simulink model "IOT_IOT"  (R2024b)
settings: Solver=VariableStepAuto  StartTime=0.0  StopTime=1  RelTol=1e-3
undefined symbols (not defined in the file): Acid, Lead, sigbuilder_block
libraries: spsBatteryLib x81, spsVoltageMeasurementLib x24, spsSeriesRLCBranchLib x23, spsIdealSwitchLib x11, slpidlib x9, spsMosfetLib x9, spsPWMGeneratorDCDCLib x7, spsPWMGenerator2LevelLib x5, spsDiodeLib x4, spsPowerLib x3, spsThreePhaseSeriesRLCLoadLib x2, spsThreePhaseVIMeasurementLib x2
(part 1 of 4)
settings Model: SimulationMode=accelerator  Creator=Jatay  LastModifiedBy=Jatay

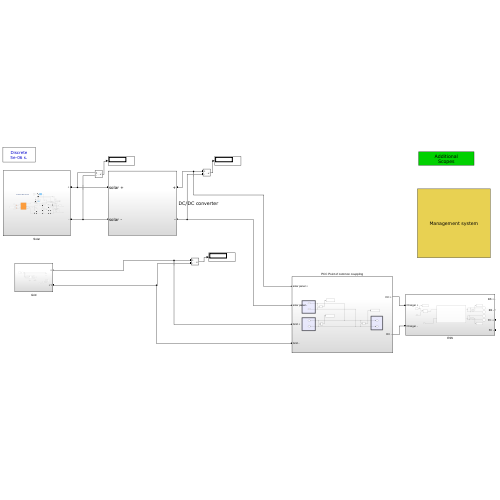
[thumbnail: Simulink's stored preview of the top-level diagram]
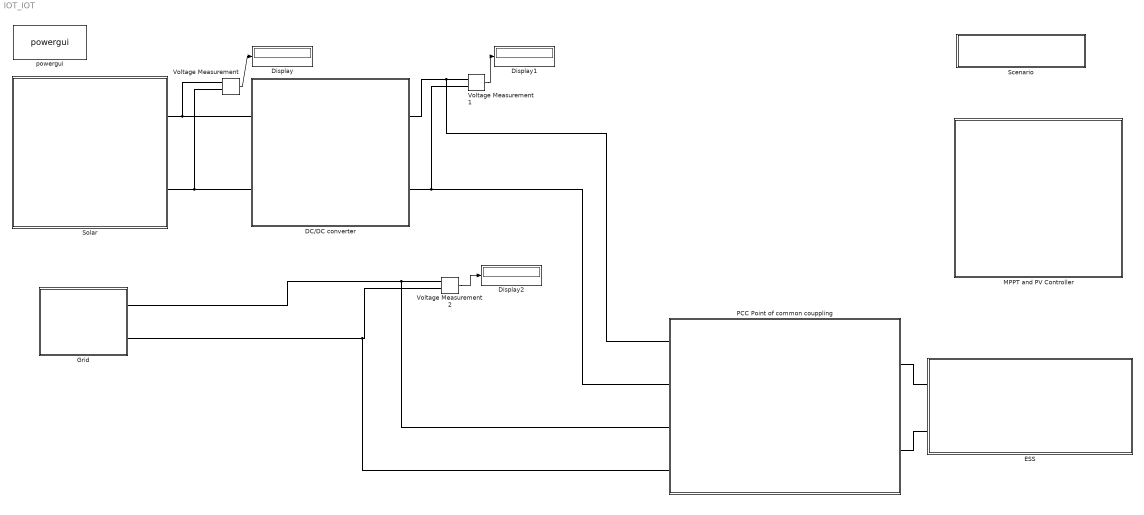
== system IOT_IOT ==
  DC/DC converter : Subsystem
  Display : Display
  Display1 : Display
  Display2 : Display
  ESS : Subsystem
  Grid : Subsystem
  MPPT and PV Controller : Subsystem
      mask Display: disp('Management system')
  PCC Point of common couppling : Subsystem
  Scenario : Subsystem
      mask Display: disp('Additional\nScopes')
  Solar : Subsystem
  Voltage Measurement : spsVoltageMeasurementLib/Voltage Measurement  PhasorSimulation=off  OutputType=Complex  PSBequivalent=0
  Voltage Measurement1 : spsVoltageMeasurementLib/Voltage Measurement  PhasorSimulation=off  OutputType=Complex  PSBequivalent=0
  Voltage Measurement2 : spsVoltageMeasurementLib/Voltage Measurement  PhasorSimulation=off  OutputType=Complex  PSBequivalent=0
  powergui : spspowerguiLib/powergui  Priority=1  SimulationMode=Discrete  SampleTime=5e-6  frequency=60  Iterations=50  frequencyindice=0  Pbase=100e6  ErrMax=1e-4  UnitsV=kV  UnitsW=MW  buscounter=0  FunctionMessages=off  echomessages=off  EnableUseOfTLC=off  CurrentSourceSwitches=off  DisableSnubberDevices=off  DisableRonSwitches=off  DisableVfSwitches=off  DisplayEquations=off  AutomaticDiscreteSolvers=off  SolverType=Tustin  Interpol=off  ExternalGateDelay=off  methode=off  Ts=0  x0status=blocks  SPID=off  SwTol=0  HookPort=off  NonlinearTolerance=1e-4  nMaxIteration=100  ContinueOnMaxIteration=off  RestoreLinks=warning  ResistiveCurrentMeasurement=off  Frange=[0:2:500]  Ylog=off  Xlog=on  ShowGrid=off  save=off  variable=ZData  structure=0  ZoomFFT=off  StartTime=0.0  cycles=1  DisplayStyle=1  fundamental=60  FreqAxis=off  MaxFrequency=1000  frequencyindicesteady=1  RmsSteady=1  display=off
  wires:
  Voltage Measurement/1 -> Display/1
  Voltage Measurement1/1 -> Display1/1
  Voltage Measurement2/1 -> Display2/1
  connections:
  Voltage Measurement1/LConn1 -- PCC Point of common couppling/LConn1 -- DC/DC converter/RConn1
  Voltage Measurement1/LConn2 -- PCC Point of common couppling/LConn2 -- DC/DC converter/RConn2
  DC/DC converter/LConn1 -- Voltage Measurement/LConn1 -- Solar/RConn1
  DC/DC converter/LConn2 -- Voltage Measurement/LConn2 -- Solar/RConn2
  Grid/RConn2 -- PCC Point of common couppling/LConn4 -- Voltage Measurement2/LConn2
  Grid/RConn1 -- PCC Point of common couppling/LConn3 -- Voltage Measurement2/LConn1
  PCC Point of common couppling/RConn1 -- ESS/LConn1
  ESS/LConn2 -- PCC Point of common couppling/RConn2

== system IOT_IOT/DC//DC converter ==
  DC - DC Converter : Subsystem
  DC bus : Subsystem
  Display1 : Display
  Voltage Measurement1 : spsVoltageMeasurementLib/Voltage Measurement  PhasorSimulation=off  OutputType=Complex  PSBequivalent=0
  Voltage Measurement2 : spsVoltageMeasurementLib/Voltage Measurement  PhasorSimulation=off  OutputType=Complex  PSBequivalent=0
  solar + : PMIOPort  Side=Left
  solar - : PMIOPort  Port=2  Side=Left
  + : PMIOPort  Port=3  Side=Right
  - : PMIOPort  Port=4  Side=Right
  tag scope: solar_controller=global
  wires:
  Voltage Measurement2/1 -> [solar_controller]
  Voltage Measurement1/1 -> Display1/1
  connections:
  DC - DC Converter/RConn1 -- DC bus/LConn1
  solar +/RConn1 -- DC - DC Converter/LConn1 -- Voltage Measurement2/LConn1
  DC - DC Converter/LConn2 -- Voltage Measurement2/LConn2 -- solar -/RConn1
  DC - DC Converter/RConn2 -- DC bus/LConn2
  DC bus/RConn2 -- -/RConn1 -- Voltage Measurement1/LConn2
  DC bus/RConn1 -- +/RConn1 -- Voltage Measurement1/LConn1

== system IOT_IOT/ESS ==
  Display : Display
  Display1 : Display
  Display2 : Display
  Ideal Switch : spsIdealSwitchLib/Ideal Switch  Ron=0.001  Lon=0  IC=0  Rs=1e5  Cs=inf  Measurements=off
  Subsystem : Subsystem
  Voltage Measurement : spsVoltageMeasurementLib/Voltage Measurement  PhasorSimulation=off  OutputType=Complex  PSBequivalent=0
  Voltage Measurement1 : spsVoltageMeasurementLib/Voltage Measurement  PhasorSimulation=off  OutputType=Complex  PSBequivalent=0
  Charger + : PMIOPort  Side=Left
  Charger - : PMIOPort  Port=2  Side=Left
  BS + : PMIOPort  Port=3  Side=Right
  BS - : PMIOPort  Port=4  Side=Right
  FC + : PMIOPort  Port=5  Side=Right
  FC - : PMIOPort  Port=6  Side=Right
  wires:
  [ss] -> Display/1, Ideal Switch/1
  Voltage Measurement/1 -> Display1/1
  Voltage Measurement1/1 -> Display2/1
  connections:
  Ideal Switch/LConn1 -- Charger +/RConn1
  Charger -/RConn1 -- Subsystem/LConn2
  Ideal Switch/RConn1 -- Subsystem/LConn1
  FC -/RConn1 -- Voltage Measurement/LConn2 -- Voltage Measurement/LConn1 -- BS -/RConn1 -- Subsystem/RConn2
  Subsystem/RConn1 -- Voltage Measurement1/LConn2 -- FC +/RConn1 -- Voltage Measurement1/LConn1 -- BS +/RConn1

== system IOT_IOT/Grid ==
  Display : Display
  Grid : spsThreePhaseSourceLib/Three-Phase Source  InternalConnection=Yg  VoltagePhases=off  Voltage=380  PhaseAngle=0  Voltage_phases=[25e3 25e3 25e3]/sqrt(3)  PhaseAngles_phases=[0 -120 +120]  Frequency=50  NonIdealSource=on  SpecifyImpedance=on  Resistance=0.8929  Inductance=16.58e-3  ShortCircuitLevel=100e6  BaseVoltage=380  XRratio=7  BusType=swing  Pref=10e3  Qref=0  Prefabc=[10e3, 10e3, 10e3]  Qrefabc=[0, 0, 0]  Qmin=-inf  Qmax=inf
  LOAD1 : spsThreePhaseSeriesRLCLoadLib/Three-Phase Series RLC Load  LConnTagsString=A|B|C  Configuration=Y (grounded)  NominalVoltage=380  Vabc=[1e3 1e3 1e3]  Vabcp=[1e3 1e3 1e3]  NominalFrequency=50  UnbalancedPower=off  ActivePower=1e3  InductivePower=0  CapacitivePower=0  Pabc=[10e3 9e3 11e3]  QLabc=[100 90 110]  QCabc=[100 90 110]  Pabcp=[10e3 9e3 11e3]  QLabcp=[100 90 110]  QCabcp=[100 90 110]  Measurements=None  LoadType=constant Z
  Measurement : spsThreePhaseVIMeasurementLib/Three-Phase V-I Measurement  VoltageMeasurement=phase-to-phase  SetLabelV=on  LabelV=Vabc_grid  Vpu=off  VpuLL=off  CurrentMeasurement=yes  SetLabelI=on  LabelI=Iabc_grid  Ipu=off  Pbase=100e6  Vbase=500e3  OutputType=Complex  PhasorSimulation=off  PSBequivalent=0
  Mux : Mux  Inputs=2
  Repeating Sequence Stair : simulink/Sources/Repeating Sequence Stair  OutValues=[0 0 1 1 0].'  tsamp=0.1  OutMin=[]  OutMax=[]  OutDataTypeStr=double  OutputDataTypeScalingMode=double  OutDataType=fixdt(0,8)  ConRadixGroup=Best Precision: Vector-wise  OutScaling=2^-12
  Scope : Scope
  Scope1 : Scope
  Scope2 : Scope  NumInputPorts=2
  V2G & G2V results : Scope  NumInputPorts=3
  Voltage Measurement : spsVoltageMeasurementLib/Voltage Measurement  PhasorSimulation=off  OutputType=Complex  PSBequivalent=0
  Wall charger Connection Box : Subsystem
  + : PMIOPort  Side=Right
  +1 : PMIOPort  Port=2  Side=Right
  tag scope: Control=global
  wires:
  [Control] -> Wall charger Connection Box/1(Control)
  Mux/1 -> V2G & G2V results/3
  [Vabc_grid] -> V2G & G2V results/1
  [Vabc_inv] -> V2G & G2V results/2
  Repeating Sequence Stair/1 -> [Control], Scope1/1
  [Vabc_inv] -> Mux/2
  [Iabc_out] -> Scope2/2
  [Iabc_inv] -> Scope/1
  [Vabc_out] -> Scope2/1
  Voltage Measurement/1 -> Display/1
  [Vabc_grid] -> Mux/1
  connections:
  Wall charger Connection Box/RConn2 -- Voltage Measurement/LConn2 -- +1/RConn1
  Grid/RConn1 -- Measurement/LConn1
  Grid/RConn3 -- Measurement/LConn3
  Wall charger Connection Box/RConn1 -- Voltage Measurement/LConn1 -- +/RConn1
  Grid/RConn2 -- Measurement/LConn2
  LOAD1/LConn3 -- Wall charger Connection Box/LConn3 -- Measurement/RConn3
  Measurement/RConn2 -- Wall charger Connection Box/LConn2 -- LOAD1/LConn2
  Measurement/RConn1 -- Wall charger Connection Box/LConn1 -- LOAD1/LConn1

== system IOT_IOT/MPPT and PV Controller ==
  Battery controller : Subsystem
  Inverter controller : Subsystem
  MMPT Controller : Subsystem
  Solar controller : Subsystem
  Swapping battery controller : Subsystem

== system IOT_IOT/PCC Point of common couppling ==
  note: ESS
  note: Grid
  note: Solar
  Display : Display
  Display1 : Display
  Display2 : Display
  Voltage Measurement : spsVoltageMeasurementLib/Voltage Measurement  PhasorSimulation=off  OutputType=Complex  PSBequivalent=0
  Voltage Measurement1 : spsVoltageMeasurementLib/Voltage Measurement  PhasorSimulation=off  OutputType=Complex  PSBequivalent=0
  Voltage Measurement2 : spsVoltageMeasurementLib/Voltage Measurement  PhasorSimulation=off  OutputType=Complex  PSBequivalent=0
  DC + : PMIOPort  Side=Right
  solar panel + : PMIOPort  Port=2  Side=Left
  solar panel - : PMIOPort  Port=3  Side=Left
  DC - : PMIOPort  Port=4  Side=Right
  Grid + : PMIOPort  Port=5  Side=Left
  Grid - : PMIOPort  Port=6  Side=Left
  wires:
  Voltage Measurement/1 -> Display/1
  Voltage Measurement1/1 -> Display1/1
  Voltage Measurement2/1 -> Display2/1
  connections:
  DC +/RConn1 -- Voltage Measurement2/LConn1 -- Voltage Measurement1/LConn1 -- Grid +/RConn1 -- Voltage Measurement/LConn1 -- solar panel +/RConn1
  solar panel -/RConn1 -- Voltage Measurement/LConn2 -- Grid -/RConn1 -- Voltage Measurement1/LConn2 -- Voltage Measurement2/LConn2 -- DC -/RConn1

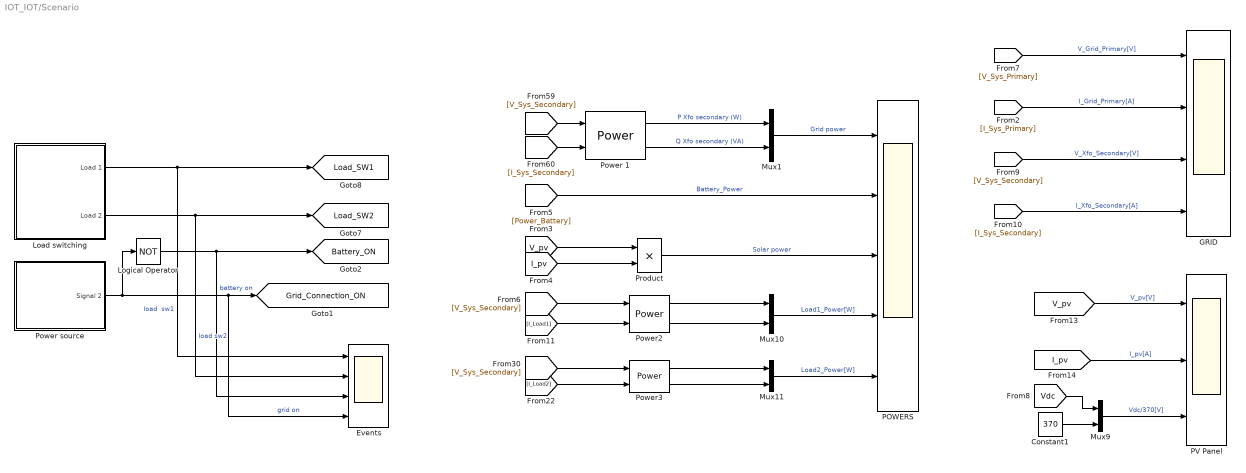
== system IOT_IOT/Scenario ==
  Constant1 : Constant  Value=370
  Events : Scope  NumInputPorts=4
  GRID : Scope  NumInputPorts=4
  Load switching : Subsystem  Tag=STV Subsys  LoadFcn=sigbuilder_block('load');  StartFcn=sigbuilder_block('start');  StopFcn=sigbuilder_block('stop');  ClipboardFcn=sigbuilder_block('clipboard');  mask(Sigbuilder block){tuvar=[0:10]}
      mask help: Simulink:masks:SigbuilderBlock_MD
      mask init:
      | if ~strcmp(get_param(bdroot(gcbh),'SimulationStatus'),'stopped') tuvar = sigbuilder_block('maskInit'); end
      settings: CopyFcn=sigbuilder_block('copy');  DeleteFcn=sigbuilder_block('delete');  ModelCloseFcn=sigbuilder_block('modelClose');  PreSaveFcn=sigbuilder_block('preSave');  PauseFcn=sigbuilder_block('pause');  ContinueFcn=sigbuilder_block('continue');  NameChangeFcn=sigbuilder_block('namechange');  OpenFcn=sigbuilder_block('open',[57 105.75 1180.5 663.75 ]);  CloseFcn=sigbuilder_block('close');
      mask Display: plot(0, 0, 100, 100,[2, 2, 32, 32, 2], [68, 8, 8, 68, 68],[32, 2], [38, 38], [32, 19, 2],[53, 60, 44], [32, 17, 17, 2],[16, 16, 31, 31]);txt = getActiveGroup(gcbh);text(2, 100, txt,'verticalAlignment', 'top');
  Logical Operator : Logic  Operator=NOT  AllPortsSameDT=off  OutDataTypeStr=boolean
  Mux{1,9..11} (4 alike) : Mux  Inputs=2
  POWERS : Scope  NumInputPorts=5
  PV Panel : Scope  NumInputPorts=3
  Power 1 : spsPowerLib/Power  Freq=60  Vinit=[1, 0]  Iinit=[1, 0]  Ts=0
  Power source : Subsystem  Tag=STV Subsys  LoadFcn=sigbuilder_block('load');  StartFcn=sigbuilder_block('start');  StopFcn=sigbuilder_block('stop');  ClipboardFcn=sigbuilder_block('clipboard');  mask(Sigbuilder block){tuvar=[0:10]}
      mask help: Simulink:masks:SigbuilderBlock_MD
      mask init:
      | if ~strcmp(get_param(bdroot(gcbh),'SimulationStatus'),'stopped') tuvar = sigbuilder_block('maskInit'); end
      settings: CopyFcn=sigbuilder_block('copy');  DeleteFcn=sigbuilder_block('delete');  ModelCloseFcn=sigbuilder_block('modelClose');  PreSaveFcn=sigbuilder_block('preSave');  PauseFcn=sigbuilder_block('pause');  ContinueFcn=sigbuilder_block('continue');  NameChangeFcn=sigbuilder_block('namechange');  OpenFcn=sigbuilder_block('open',[436.966 199.241 549.931 400.345 ]);  CloseFcn=sigbuilder_block('close');
      mask Display: plot(0, 0, 100, 100,[2, 2, 32, 32, 2], [68, 8, 8, 68, 68],[32, 2], [38, 38], [32, 19, 2],[53, 60, 44], [32, 17, 17, 2],[16, 16, 31, 31]);txt = getActiveGroup(gcbh);text(2, 100, txt,'verticalAlignment', 'top');
  Power2 : spsPowerLib/Power  Freq=60  Vinit=[1, 0]  Iinit=[1, 0]  Ts=0
  Power3 : spsPowerLib/Power  Freq=60  Vinit=[1, 0]  Iinit=[1, 0]  Ts=0
  Product : Product  RndMeth=Zero
  tag scope: Battery_ON=global, Grid_Connection_ON=global, Load_SW1=global, Load_SW2=global
  wires:
  Load switching/2(Load 2) -> [Load_SW2], Events/2  "load sw2"
  Logical Operator/1 -> Events/3, [Battery_ON]  "battery on"
  Power source/1(Signal 2) -> Events/4, [Grid_Connection_ON], Logical Operator/1  "grid on"
  Load switching/1(Load 1) -> [Load_SW1], Events/1  "load  sw1"
  [Vdc] -> Mux9/1
  Constant1/1 -> Mux9/2
  Mux9/1 -> PV Panel/3  "Vdc/370[V]"
  [V_Sys_Primary] -> GRID/1  "V_Grid_Primary[V]"
  [I_Sys_Primary] -> GRID/2  "I_Grid_Primary[A]"
  [V_Sys_Secondary] -> GRID/3  "V_Xfo_Secondary[V]"
  [I_Sys_Secondary] -> GRID/4  "I_Xfo_Secondary[A]"
  [V_pv] -> PV Panel/1  "V_pv[V]"
  [I_pv] -> PV Panel/2  "I_pv[A]"
  [V_pv] -> Product/1
  [I_pv] -> Product/2
  Product/1 -> POWERS/3  "Solar power"
  [Power_Battery] -> POWERS/2  "Battery_Power"
  [V_Sys_Secondary] -> Power 1/1
  [I_Sys_Secondary] -> Power 1/2
  [V_Sys_Secondary] -> Power2/1
  [I_Load1] -> Power2/2
  Mux10/1 -> POWERS/4  "Load1_Power[W]"
  [V_Sys_Secondary] -> Power3/1
  [I_Load2] -> Power3/2
  Mux11/1 -> POWERS/5  "Load2_Power[W]"
  Power2/1 -> Mux10/1
  Power2/2 -> Mux10/2
  Power3/1 -> Mux11/1
  Power3/2 -> Mux11/2
  Mux1/1 -> POWERS/1  "Grid power"
  Power 1/1 -> Mux1/1  "P Xfo secondary (W)"
  Power 1/2 -> Mux1/2  "Q Xfo secondary (VA)"

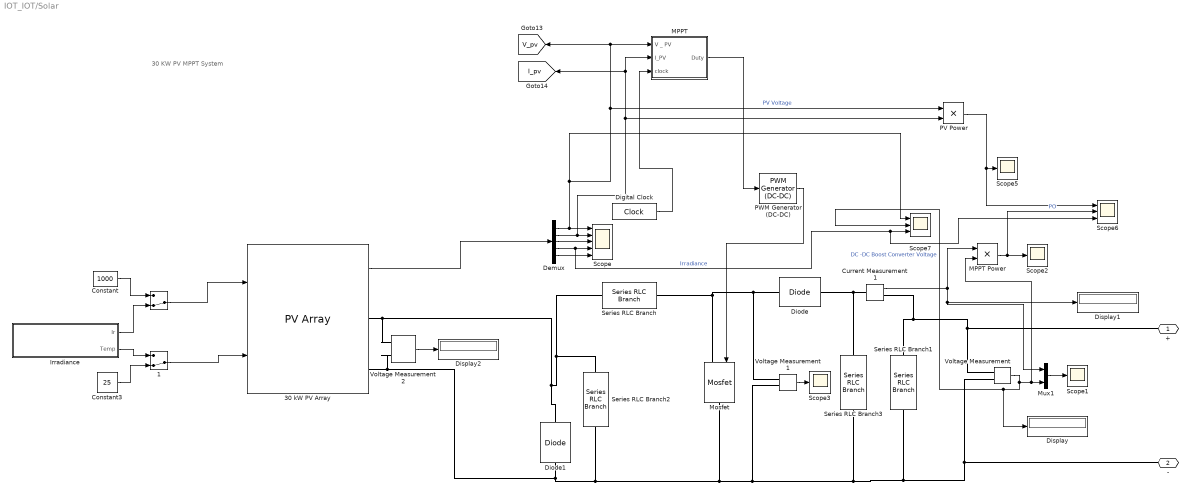
== system IOT_IOT/Solar ==
  note: 30 KW PV MPPT System
  "      " : ManualSwitch  CurrentSetting=0
  "      1" : ManualSwitch  CurrentSetting=0
  30 kW PV Array : spsPVArrayLib/PV Array  Npar=15  Nser=10  PlotType=array @ 1000 W/m2 & specified temperatures  S_vec="[ 1000  500  100 ]"  Temp_C_vec="[ 45 25  ]"  ModuleName=User-defined  PlotWhenSelected=off  Pm=213.15  Ncell=60  Voc=48  Isc=7.84  Vm=29  Im=7.35  beta_Voc_pc=-0.36099  alpha_Isc_pc=0.102  beta_Voc=-0.17328  alpha_Isc=0.0079968  IL=8.2285  I0=2.9956e-10  nI=1.2955  Rsh=7353.5939  Rs=2.0228  RobustModel=off  RobustCellTemperature=25  BAL=on  Tc=1e-6  Tfilter=5e-5
  Constant : Constant  Value=1000
  Constant3 : Constant  Value=25
  Current Measurement1 : spsCurrentMeasurementLib/Current Measurement  PhasorSimulation=off  OutputType=Complex  PSBequivalent=0
  Demux : Demux  Outputs=5
  Digital Clock : DigitalClock  SampleTime=0.001
  Diode : spsDiodeLib/Diode  Ron=0.5  Lon=0  Vf=0.7  IC=0  UseSnubber=0  Rs=1e5  Cs=250e-9  Measurements=off
  Diode1 : spsDiodeLib/Diode  Ron=0.5  Lon=0  Vf=0.7  IC=0  UseSnubber=0  Rs=1e5  Cs=250e-9  Measurements=off
  Display : Display
  Display1 : Display
  Display2 : Display
  "Irradiance " : Subsystem  Tag=STV Subsys  LoadFcn=sigbuilder_block('load');  StartFcn=sigbuilder_block('start');  StopFcn=sigbuilder_block('stop');  ClipboardFcn=sigbuilder_block('clipboard');  mask(Sigbuilder block){tuvar=[0:10]}
      mask help: Sigbuilder GUI
      mask init:
      | if ~strcmp(get_param(bdroot(gcbh),'SimulationStatus'),'stopped') tuvar = sigbuilder_block('maskInit'); end
      settings: CopyFcn=sigbuilder_block('copy');  DeleteFcn=sigbuilder_block('delete');  ModelCloseFcn=sigbuilder_block('modelClose');  PreSaveFcn=sigbuilder_block('preSave');  PauseFcn=sigbuilder_block('pause')  ContinueFcn=sigbuilder_block('continue')  NameChangeFcn=sigbuilder_block('namechange');  OpenFcn=sigbuilder_block('open',[5.4 30 1141.2 507.6 ]);  CloseFcn=sigbuilder_block('close');
      mask Display: plot(0, 0, 100, 100,[2, 2, 32, 32, 2], [68, 8, 8, 68, 68],[32, 2], [38, 38], [32, 19, 2],[53, 60, 44], [32, 17, 17, 2],[16, 16, 31, 31]);txt = getActiveGroup(gcbh);text(2, 100, txt,'verticalAlignment', 'top');
  MPPT : Subsystem
  MPPT Power : Product
  Mosfet : spsMosfetLib/Mosfet  Ron=0.1  Lon=0  Rd=0.01  Vfd=0.7  IC=0  Rs=1e5  Cs=inf  Measurements=off
  Mux1 : Mux  Inputs=2
  PV Power : Product
  PWM Generator (DC-DC) : spsPWMGeneratorDCDCLib/PWM Generator (DC-DC)  Fsw=1500  Ts=0
  Scope : Scope  NumInputPorts=5
  Scope{1..3,5} (4 alike) : Scope
  Scope6 : Scope  NumInputPorts=3
  Scope7 : Scope  NumInputPorts=3
  Series RLC Branch : spsSeriesRLCBranchLib/Series RLC Branch  LConnTagsString=__new0  RConnTagsString=__new0  BranchType=L  Resistance=0.001  Inductance=0.4e-1  SetiL0=off  InitialCurrent=0  Capacitance=1e-6  Setx0=off  InitialVoltage=0  Measurements=None
  Series RLC Branch1 : spsSeriesRLCBranchLib/Series RLC Branch  LConnTagsString=__new0  RConnTagsString=__new0  BranchType=R  Resistance=11  Inductance=0.1  SetiL0=off  InitialCurrent=0  Capacitance=100e-6  Setx0=off  InitialVoltage=0  Measurements=None
  Series RLC Branch2 : spsSeriesRLCBranchLib/Series RLC Branch  LConnTagsString=__new0  RConnTagsString=__new0  BranchType=C  Resistance=6  Inductance=0.1  SetiL0=off  InitialCurrent=0  Capacitance=700e-5  Setx0=off  InitialVoltage=0  Measurements=None
  Series RLC Branch3 : spsSeriesRLCBranchLib/Series RLC Branch  LConnTagsString=__new0  RConnTagsString=__new0  BranchType=C  Resistance=6  Inductance=0.1  SetiL0=off  InitialCurrent=0  Capacitance=1000e-5  Setx0=off  InitialVoltage=0  Measurements=None
  Voltage Measurement : spsVoltageMeasurementLib/Voltage Measurement  PhasorSimulation=off  OutputType=Complex  PSBequivalent=0
  Voltage Measurement1 : spsVoltageMeasurementLib/Voltage Measurement  PhasorSimulation=off  OutputType=Complex  PSBequivalent=0
  Voltage Measurement2 : spsVoltageMeasurementLib/Voltage Measurement  PhasorSimulation=off  OutputType=Complex  PSBequivalent=0
  + : PMIOPort  Side=Right
  - : PMIOPort  Port=2  Side=Right
  tag scope: I_pv=global, V_pv=global
  wires:
  Voltage Measurement/1 -> MPPT Power/2, Mux1/2, Display/1, Scope7/2  "DC -DC Boost Converter Voltage"
  PWM Generator (DC-DC)/1 -> Mosfet/1
  Demux/1 -> Scope7/1, PV Power/1, [V_pv], MPPT/1("V _ PV "), Scope/1  "PV Voltage"
  Mux1/1 -> Scope1/1
  MPPT Power/1 -> Scope6/2, Scope2/1  "PO"
  Demux/2 -> PV Power/2, [I_pv], MPPT/2(I_PV), Scope/2
  Current Measurement1/1 -> MPPT Power/1, Display1/1, Mux1/1
  Voltage Measurement1/1 -> Scope3/1
  Demux/3 -> Scope/3
  Demux/4 -> Scope6/3, Scope7/3, Scope/4  "Irradiance"
  Digital Clock/1 -> MPPT/3(clock)
  MPPT/1(Duty) -> PWM Generator (DC-DC)/1
  PV Power/1 -> Scope6/1, Scope5/1
  Demux/5 -> Scope/5
  "Irradiance "/2(Temp) -> "      1"/1
  Constant3/1 -> "      1"/2
  "Irradiance "/1(Ir) -> "      "/2
  Constant/1 -> "      "/1
  "      "/1 -> 30 kW PV Array/1
  "      1"/1 -> 30 kW PV Array/2
  30 kW PV Array/1 -> Demux/1
  Voltage Measurement2/1 -> Display2/1
  connections:
  Voltage Measurement/LConn2 -- Voltage Measurement2/LConn2 -- 30 kW PV Array/RConn2 -- Diode1/LConn1 -- Series RLC Branch2/RConn1 -- Mosfet/RConn1 -- Voltage Measurement1/LConn2 -- Series RLC Branch3/RConn1 -- Series RLC Branch1/RConn1 -- -/RConn1
  Current Measurement1/RConn1 -- Series RLC Branch1/LConn1 -- Voltage Measurement/LConn1 -- +/RConn1
  Diode/RConn1 -- Series RLC Branch3/LConn1 -- Current Measurement1/LConn1
  Voltage Measurement1/LConn1 -- Series RLC Branch/RConn1 -- Mosfet/LConn1 -- Diode/LConn1
  Series RLC Branch2/LConn1 -- Voltage Measurement2/LConn1 -- 30 kW PV Array/RConn1 -- Diode1/RConn1 -- Series RLC Branch/LConn1

== system IOT_IOT/DC//DC converter/DC - DC Converter ==
  C : spsSeriesRLCBranchLib/Series RLC Branch  LConnTagsString=__new0  RConnTagsString=__new0  BranchType=C  Resistance=0.01  Inductance=1e-3  SetiL0=off  InitialCurrent=0  Capacitance=1000e-6  Setx0=on  InitialVoltage=200  Measurements=None
  Diode : spsDiodeLib/Diode  Ron=0.001  Lon=0  Vf=1.1  IC=0  UseSnubber=off  Rs=500  Cs=250e-9  Measurements=off
  Diode2 : spsDiodeLib/Diode  Ron=0.001  Lon=0  Vf=0.7  IC=0  UseSnubber=off  Rs=500  Cs=250e-9  Measurements=off
  IGBT : spsIGBTLib/IGBT  Ron=0.001  Lon=0  Vf=1.1  Tf=1e-6  Tt=2e-6  IC=0  Rs=1e5  Cs=inf  Measurements=off
  RL : spsSeriesRLCBranchLib/Series RLC Branch  LConnTagsString=__new0  RConnTagsString=__new0  BranchType=RL  Resistance=0.05  Inductance=470e-6  SetiL0=off  InitialCurrent=0  Capacitance=1e-6  Setx0=off  InitialVoltage=0  Measurements=None
  DC + : PMIOPort  Side=Right
  solar panel + : PMIOPort  Port=2  Side=Left
  solar panel - : PMIOPort  Port=3  Side=Left
  DC - : PMIOPort  Port=4  Side=Right
  wires:
  [Pulse_PV] -> IGBT/1
  connections:
  Diode/RConn1 -- DC +/RConn1
  Diode2/RConn1 -- C/LConn1 -- RL/LConn1
  Diode/LConn1 -- RL/RConn1 -- IGBT/LConn1
  solar panel +/RConn1 -- Diode2/LConn1
  C/RConn1 -- solar panel -/RConn1 -- DC -/RConn1 -- IGBT/RConn1

== system IOT_IOT/DC//DC converter/DC bus ==
  1 ohm 2000uH : spsSeriesRLCBranchLib/Series RLC Branch  LConnTagsString=__new0  RConnTagsString=__new0  BranchType=RC  Resistance=1  Inductance=0  SetiL0=off  InitialCurrent=0  Capacitance=2000e-6  Setx0=on  InitialVoltage=370  Measurements=None
  RL + : spsSeriesRLCBranchLib/Series RLC Branch  LConnTagsString=__new0  RConnTagsString=__new0  BranchType=RL  Resistance=0.05  Inductance=470e-6  SetiL0=off  InitialCurrent=0  Capacitance=1e-6  Setx0=off  InitialVoltage=0  Measurements=None
  RL - : spsSeriesRLCBranchLib/Series RLC Branch  LConnTagsString=__new0  RConnTagsString=__new0  BranchType=RL  Resistance=0.05  Inductance=470e-6  SetiL0=off  InitialCurrent=0  Capacitance=1e-6  Setx0=off  InitialVoltage=0  Measurements=None
  Transfer Fcn : TransferFcn  Denominator=[1e-4 1]
  V : spsVoltageMeasurementLib/Voltage Measurement  PhasorSimulation=off  OutputType=Complex  PSBequivalent=0
  left + : PMIOPort  Side=Left
  left - : PMIOPort  Port=2  Side=Left
  right + : PMIOPort  Port=3  Side=Right
  right - : PMIOPort  Port=4  Side=Right
  tag scope: Vdc=global
  wires:
  V/1 -> Transfer Fcn/1
  Transfer Fcn/1 -> [Vdc]
  connections:
  RL +/RConn1 -- 1 ohm 2000uH/LConn1 -- right +/RConn1 -- V/LConn1
  RL -/RConn1 -- 1 ohm 2000uH/RConn1 -- right -/RConn1 -- V/LConn2
  left +/RConn1 -- RL +/LConn1
  left -/RConn1 -- RL -/LConn1

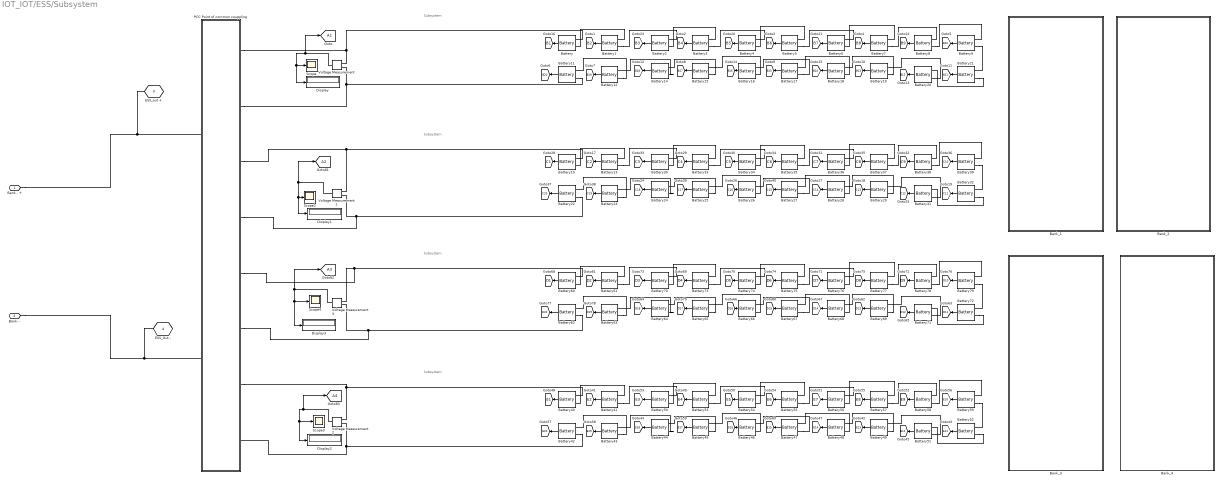
== system IOT_IOT/ESS/Subsystem ==
  note: Subsystem
  note: Subsystem
  note: Subsystem
  note: Subsystem
  Bank_1 : Subsystem
  Bank_2 : Subsystem
  Bank_3 : Subsystem
  Bank_4 : Subsystem
  Battery{,1..79} (80 alike) : spsBatteryLib/Battery  BatType=Lead-Acid  NomV=12  NomQ=100  SOC=80  Batt_Tr=10  PresetModel=on  MaxQ=104.1667  MinV=9  FullV=13.0658  Dis_rate=20  R=0.0012  Normal_OP=31.0278  expZone="[12.2171     0.333333]"
  Display{,1..3} (4 alike) : Display
  PCC Point of common couppling : Subsystem
  Scope{,2..4} (4 alike) : Scope
  Voltage Measurement{,1..3} (4 alike) : spsVoltageMeasurementLib/Voltage Measurement  PhasorSimulation=off  OutputType=Complex  PSBequivalent=0
  Bank - + : PMIOPort  Side=Left
  Bank- - : PMIOPort  Port=2  Side=Left
  ESS_out + : PMIOPort  Port=3  Side=Right
  ESS_Out - : PMIOPort  Port=4  Side=Right
  tag scope: A1=global, A2=global, A3=global, A4=global, B10=global, B11=global, B12=global, B13=global, B14=global, B15=global, B16=global, B17=global, B18=global, B19=global, B1=global, B20=global, B2=global, B3=global, B4=global, B5=global, B6=global, B7=global, B8=global, B9=global, C10=global, C11=global, C12=global, C13=global, C14=global, C15=global, C16=global, C17=global, C18=global, C19=global, C1=global, C20=global, C2=global, C3=global, C4=global, C5=global, C6=global, C7=global, C8=global, C9=global, D10=global, D11=global, D12=global, D13=global, D14=global, D15=global, D16=global, D17=global, D18=global, D19=global, D1=global, D20=global, D2=global, D3=global, D4=global, D5=global, D6=global, D7=global, D8=global, D9=global, E10=global, E11=global, E12=global, E13=global, E14=global, E15=global, E16=global, E17=global, E18=global, E19=global, E1=global, E20=global, E2=global, E3=global, E4=global, E5=global, E6=global, E7=global, E8=global, E9=global
  wires:
  Voltage Measurement/1 -> [A1], Scope/1, Display/1
  Battery1/1 -> [B2]
  Battery5/1 -> [B6]
  Battery25/1 -> [C17]
  Battery53/1 -> [E4]
  Battery20/1 -> [B12]
  Battery34/1 -> [C5]
  Battery28/1 -> [C14]
  Battery4/1 -> [B5]
  Battery45/1 -> [E17]
  Battery56/1 -> [E7]
  Voltage Measurement2/1 -> [A4], Scope3/1, Display2/1
  Battery16/1 -> [B16]
  Battery2/1 -> [B3]
  Battery18/1 -> [B14]
  Battery14/1 -> [B18]
  Voltage Measurement3/1 -> [A3], Display3/1, Scope4/1
  Battery8/1 -> [B9]
  Battery6/1 -> [B7]
  Battery17/1 -> [B15]
  Battery79/1 -> [D10]
  Battery65/1 -> [D17]
  Battery24/1 -> [C18]
  Battery9/1 -> [B10]
  Battery12/1 -> [B19]
  Battery61/1 -> [D2]
  Battery15/1 -> [B17]
  Battery21/1 -> [B11]
  Battery57/1 -> [E8]
  Battery11/1 -> [B20]
  Battery10/1 -> [C1]
  Battery64/1 -> [D18]
  Battery19/1 -> [B13]
  Battery73/1 -> [D4]
  Battery3/1 -> [B4]
  Battery41/1 -> [E2]
  Battery7/1 -> [B8]
  Battery49/1 -> [E13]
  Battery55/1 -> [E6]
  Battery66/1 -> [D16]
  Battery44/1 -> [E18]
  Battery58/1 -> [E9]
  Battery74/1 -> [D5]
  Battery42/1 -> [E20]
  Battery27/1 -> [C15]
  Battery43/1 -> [E19]
  Battery54/1 -> [E5]
  Battery48/1 -> [E14]
  Battery47/1 -> [E15]
  Battery13/1 -> [C2]
  Battery52/1 -> [E11]
  Battery59/1 -> [E10]
  Battery51/1 -> [E12]
  Battery/1 -> [B1]
  Battery50/1 -> [E3]
  Battery40/1 -> [E1]
  Battery46/1 -> [E16]
  Voltage Measurement1/1 -> [A2], Display1/1, Scope2/1
  Battery63/1 -> [D19]
  Battery38/1 -> [C9]
  Battery22/1 -> [C20]
  Battery39/1 -> [C10]
  Battery71/1 -> [D12]
  Battery32/1 -> [C11]
  Battery37/1 -> [C8]
  Battery33/1 -> [C4]
  Battery60/1 -> [D1]
  Battery35/1 -> [C6]
  Battery23/1 -> [C19]
  Battery29/1 -> [C13]
  Battery69/1 -> [D13]
  Battery31/1 -> [C12]
  Battery36/1 -> [C7]
  Battery30/1 -> [C3]
  Battery26/1 -> [C16]
  Battery70/1 -> [D3]
  Battery68/1 -> [D14]
  Battery75/1 -> [D6]
  Battery72/1 -> [D11]
  Battery62/1 -> [D20]
  Battery77/1 -> [D8]
  Battery67/1 -> [D15]
  Battery76/1 -> [D7]
  Battery78/1 -> [D9]
  connections:
  Battery61/LConn2 -- Battery70/LConn1
  Battery7/LConn2 -- Battery8/LConn1
  Battery54/LConn2 -- Battery55/LConn1
  Battery63/LConn2 -- Battery62/LConn1
  Voltage Measurement3/LConn2 -- Battery62/LConn2 -- PCC Point of common couppling/LConn6
  Battery20/LConn2 -- Battery19/LConn1
  Battery9/LConn2 -- Battery21/LConn1
  Battery56/LConn2 -- Battery57/LConn1
  Battery43/LConn2 -- Battery42/LConn1
  Battery/LConn1 -- PCC Point of common couppling/LConn1 -- Voltage Measurement/LConn1
  Battery40/LConn1 -- Voltage Measurement2/LConn1 -- PCC Point of common couppling/LConn7
  PCC Point of common couppling/LConn2 -- Battery11/LConn2 -- Voltage Measurement/LConn2
  Voltage Measurement3/LConn1 -- Battery60/LConn1 -- PCC Point of common couppling/LConn5
  Battery68/LConn2 -- Battery67/LConn1
  Battery2/LConn2 -- Battery3/LConn1
  Battery13/LConn2 -- Battery30/LConn1
  Battery39/LConn2 -- Battery32/LConn1
  Battery15/LConn2 -- Battery14/LConn1
  Battery16/LConn2 -- Battery15/LConn1
  Battery42/LConn2 -- Voltage Measurement2/LConn2 -- PCC Point of common couppling/LConn8
  Battery52/LConn2 -- Battery51/LConn1
  Battery14/LConn2 -- Battery12/LConn1
  Battery21/LConn2 -- Battery20/LConn1
  Battery6/LConn2 -- Battery7/LConn1
  Battery12/LConn2 -- Battery11/LConn1
  Battery18/LConn2 -- Battery17/LConn1
  Battery17/LConn2 -- Battery16/LConn1
  Battery3/LConn2 -- Battery4/LConn1
  Battery19/LConn2 -- Battery18/LConn1
  Battery53/LConn2 -- Battery54/LConn1
  Battery8/LConn2 -- Battery9/LConn1
  Battery26/LConn2 -- Battery25/LConn1
  Battery1/LConn2 -- Battery2/LConn1
  Battery60/LConn2 -- Battery61/LConn1
  Battery69/LConn2 -- Battery68/LConn1
  Battery50/LConn2 -- Battery53/LConn1
  Battery4/LConn2 -- Battery5/LConn1
  Battery5/LConn2 -- Battery6/LConn1
  Battery/LConn2 -- Battery1/LConn1
  Battery41/LConn2 -- Battery50/LConn1
  Battery49/LConn2 -- Battery48/LConn1
  Battery58/LConn2 -- Battery59/LConn1
  Battery48/LConn2 -- Battery47/LConn1
  Battery57/LConn2 -- Battery58/LConn1
  Battery55/LConn2 -- Battery56/LConn1
  Battery45/LConn2 -- Battery44/LConn1
  Battery40/LConn2 -- Battery41/LConn1
  Battery46/LConn2 -- Battery45/LConn1
  Battery59/LConn2 -- Battery52/LConn1
  Battery44/LConn2 -- Battery43/LConn1
  Battery76/LConn2 -- Battery77/LConn1
  Battery51/LConn2 -- Battery49/LConn1
  Battery47/LConn2 -- Battery46/LConn1
  Battery23/LConn2 -- Battery22/LConn1
  Battery10/LConn1 -- Voltage Measurement1/LConn1 -- PCC Point of common couppling/LConn3
  Battery25/LConn2 -- Battery24/LConn1
  Battery70/LConn2 -- Battery73/LConn1
  Battery10/LConn2 -- Battery13/LConn1
  Battery72/LConn2 -- Battery71/LConn1
  Battery28/LConn2 -- Battery27/LConn1
  Battery73/LConn2 -- Battery74/LConn1
  Battery74/LConn2 -- Battery75/LConn1
  Battery29/LConn2 -- Battery28/LConn1
  Battery33/LConn2 -- Battery34/LConn1
  Battery32/LConn2 -- Battery31/LConn1
  Voltage Measurement1/LConn2 -- Battery22/LConn2 -- PCC Point of common couppling/LConn4
  Battery30/LConn2 -- Battery33/LConn1
  Battery34/LConn2 -- Battery35/LConn1
  Battery38/LConn2 -- Battery39/LConn1
  Battery35/LConn2 -- Battery36/LConn1
  Battery24/LConn2 -- Battery23/LConn1
  Battery31/LConn2 -- Battery29/LConn1
  Battery36/LConn2 -- Battery37/LConn1
  Battery66/LConn2 -- Battery65/LConn1
  Battery37/LConn2 -- Battery38/LConn1
  Battery79/LConn2 -- Battery72/LConn1
  Battery27/LConn2 -- Battery26/LConn1
  Battery67/LConn2 -- Battery66/LConn1
  Battery77/LConn2 -- Battery78/LConn1
  Battery65/LConn2 -- Battery64/LConn1
  Battery78/LConn2 -- Battery79/LConn1
  Battery71/LConn2 -- Battery69/LConn1
  Battery64/LConn2 -- Battery63/LConn1
  Battery75/LConn2 -- Battery76/LConn1
  Bank - +/RConn1 -- ESS_out +/RConn1 -- PCC Point of common couppling/RConn1
  Bank- -/RConn1 -- ESS_Out -/RConn1 -- PCC Point of common couppling/RConn2

== system IOT_IOT/Grid/Wall charger Connection Box ==
  Control : Inport
  Battery Switching Control : Subsystem
      settings: PortSchema="{\"entries\":[{\"content\":{\"sides\":[{\"content\":{\"connectorIds\":[\"LConn1\",\"LConn2\",\"LConn3\",\"LConn4\"]},\"type\":\"ConnectorPlacement.EquallySpacedRectSide\",\"uuid\":\"597ce45f-d2da-489f-9702-c83ae9b1152a\"},{\"content\":{\"connectorIds\":[\"In1\",\"RConn1\",\"RConn2\"],\"side\":\"RIGHT\"},\"type\":\"ConnectorPlacement.EquallySpacedRectSide\",\"uuid\":\"90ab1945-2787-45d6-b647-1c8eb49fe34d\"},{\"content\":{\"connectorIds\":[],\"side\":\"TOP\"},\"type\":\"ConnectorPlacement.EquallySpacedRectSide\",\"uuid\":\"5514c8fd-a1bb-4ed7-b1c0-08bce6a0e9e5\"}]},\"type\":\"ConnectorPlacement.EquallySpacedConnector\",\"uuid\":\"b6d566cb-31ba-40ab-ae9a-003997b713cb\"}],\"packageUris\":[\"http://schema.mathworks.com/mf0/Connector/R2020b\"],\"version\":\"1.0\"}"
  Buck-Boost Converter : Subsystem
  Connection Control : Subsystem
      settings: PortSchema="{\"entries\":[{\"content\":{\"sides\":[{\"content\":{\"connectorIds\":[\"LConn1\",\"LConn2\",\"LConn3\"]},\"type\":\"ConnectorPlacement.EquallySpacedRectSide\",\"uuid\":\"27ebf5cb-61b2-431e-8de2-c9344a0dfca5\"},{\"content\":{\"connectorIds\":[\"In1\",\"RConn1\",\"RConn2\",\"RConn3\",\"RConn4\",\"RConn5\",\"RConn6\"],\"side\":\"RIGHT\"},\"type\":\"ConnectorPlacement.EquallySpacedRectSide\",\"uuid\":\"2438100a-e43b-42f7-afa1-1af449516139\"},{\"content\":{\"connectorIds\":[],\"side\":\"TOP\"},\"type\":\"ConnectorPlacement.EquallySpacedRectSide\",\"uuid\":\"dcfa608d-f6dc-42e3-abf8-45a08af22825\"}]},\"type\":\"ConnectorPlacement.EquallySpacedConnector\",\"uuid\":\"5f0f36e8-f735-4489-a6f2-39fec655b509\"}],\"packageUris\":[\"http://schema.mathworks.com/mf0/Connector/R2020b\"],\"version\":\"1.0\"}"
  DC-AC / AC-DC Converter : Subsystem
  DC-DC converter with battery controller : Subsystem
  Grid_R : PMIOPort  Side=Left
  Grid_Y : PMIOPort  Port=2  Side=Left
  Grid_B : PMIOPort  Port=3  Side=Left
  Vehicle+ : PMIOPort  Port=4  Side=Right
  Vehicle- : PMIOPort  Port=5  Side=Right
  wires:
  Control/1 -> Connection Control/1(Control), Battery Switching Control/1(Control)
  connections:
  DC-AC / AC-DC Converter/LConn5 -- Connection Control/RConn5
  DC-AC / AC-DC Converter/LConn2 -- Connection Control/RConn2
  DC-DC converter with battery controller/RConn3 -- Battery Switching Control/LConn3
  Buck-Boost Converter/RConn2 -- DC-DC converter with battery controller/LConn2
  Grid_B/RConn1 -- Connection Control/LConn3
  DC-AC / AC-DC Converter/RConn3 -- Buck-Boost Converter/LConn3
  Grid_R/RConn1 -- Connection Control/LConn1
  DC-AC / AC-DC Converter/LConn1 -- Connection Control/RConn1
  Vehicle-/RConn1 -- Battery Switching Control/RConn2
  Vehicle+/RConn1 -- Battery Switching Control/RConn1
  Buck-Boost Converter/RConn4 -- DC-DC converter with battery controller/LConn4
  Grid_Y/RConn1 -- Connection Control/LConn2
  DC-AC / AC-DC Converter/LConn4 -- Connection Control/RConn4
  DC-DC converter with battery controller/RConn2 -- Battery Switching Control/LConn2
  DC-DC converter with battery controller/RConn1 -- Battery Switching Control/LConn1
  DC-DC converter with battery controller/RConn4 -- Battery Switching Control/LConn4
  Buck-Boost Converter/RConn1 -- DC-DC converter with battery controller/LConn1
  Buck-Boost Converter/LConn2 -- DC-AC / AC-DC Converter/RConn2
  DC-AC / AC-DC Converter/LConn3 -- Connection Control/RConn3
  DC-AC / AC-DC Converter/RConn1 -- Buck-Boost Converter/LConn1
  DC-AC / AC-DC Converter/RConn4 -- Buck-Boost Converter/LConn4
  Buck-Boost Converter/RConn3 -- DC-DC converter with battery controller/LConn3
  Connection Control/RConn6 -- DC-AC / AC-DC Converter/LConn6

== system IOT_IOT/MPPT and PV Controller/Battery controller ==
  Battery Controller : Subsystem
  Constant3 : Constant  Value=370
  PWM Controller 2 : Subsystem
  Transfer Fcn : TransferFcn  Denominator=[1e-2 1]
  Transfer Fcn2 : TransferFcn  Denominator=[1e-5 1]
  Transfer Fcn3 : TransferFcn  Denominator=[0.01 1]
  tag scope: G1_B=global, G2_B=global, Pulse_B=global
  wires:
  Transfer Fcn2/1 -> Battery Controller/3(I_bt)
  Transfer Fcn/1 -> Battery Controller/1(V_Dc)
  [Battery_ON] -> PWM Controller 2/Enable
  [Vdc] -> Transfer Fcn3/1
  [Vdc] -> Transfer Fcn/1
  Constant3/1 -> Battery Controller/2(370)
  [Ibt] -> Transfer Fcn2/1
  PWM Controller 2/1(Pulse) -> [Pulse_B]
  Battery Controller/1(Pulse 1) -> [G2_B]
  Transfer Fcn3/1 -> PWM Controller 2/1(Vdc)
  Battery Controller/2(Pulse 2) -> [G1_B]

== system IOT_IOT/MPPT and PV Controller/Inverter controller ==
  Constant1 : Constant  Value=370
  Inverter Controller : Subsystem
  Transfer Fcn1 : TransferFcn  Denominator=[1e-5 1]
  Transfer Fcn8 : TransferFcn  Denominator=[1e-5 1]
  tag scope: Pulse_UI=global
  wires:
  Inverter Controller/1(Pulse) -> [Pulse_UI]
  Constant1/1 -> Inverter Controller/2(370)
  [I_Sys_Secondary] -> Transfer Fcn1/1
  Transfer Fcn1/1 -> Inverter Controller/4(I_Sys_Secondary)
  [Grid_Connection_ON] -> Inverter Controller/Enable
  [V_Sys_Secondary] -> Inverter Controller/3(V_Sys_Secondary)
  [Vdc] -> Transfer Fcn8/1
  Transfer Fcn8/1 -> Inverter Controller/1(V_Dc)

== system IOT_IOT/MPPT and PV Controller/MMPT Controller ==
  MPPT Controller : Stateflow chart  TreatAsAtomicUnit=on
  PV Controller : Subsystem
  Transfer Fcn5 : TransferFcn  Denominator=[1e-5 1]
  Transfer Fcn6 : TransferFcn  Denominator=[1e-5 1]
  tag scope: Pulse_PV=global
  wires:
  Transfer Fcn6/1 -> MPPT Controller/2(I_pv), PV Controller/2(I_pv)
  PV Controller/1(Pulse) -> [Pulse_PV]
  [V_pv] -> Transfer Fcn5/1
  Transfer Fcn5/1 -> MPPT Controller/1(V_pv), PV Controller/1(V_pv)
  [I_pv] -> Transfer Fcn6/1
  MPPT Controller/1(Vref) -> PV Controller/3(Vref)

== system IOT_IOT/MPPT and PV Controller/Solar controller ==
  Constant1 : Constant  Value=0
  Constant2 : Constant
  Display2 : Display
  Display3 : Display
  Switch : Switch  Threshold=150  SaturateOnIntegerOverflow=off  InputSameDT=off
  tag scope: ss=global
  wires:
  Constant2/1 -> Switch/1
  Switch/1 -> Display2/1, [ss]
  Constant1/1 -> Switch/3
  [solar_controller] -> Display3/1, Switch/2

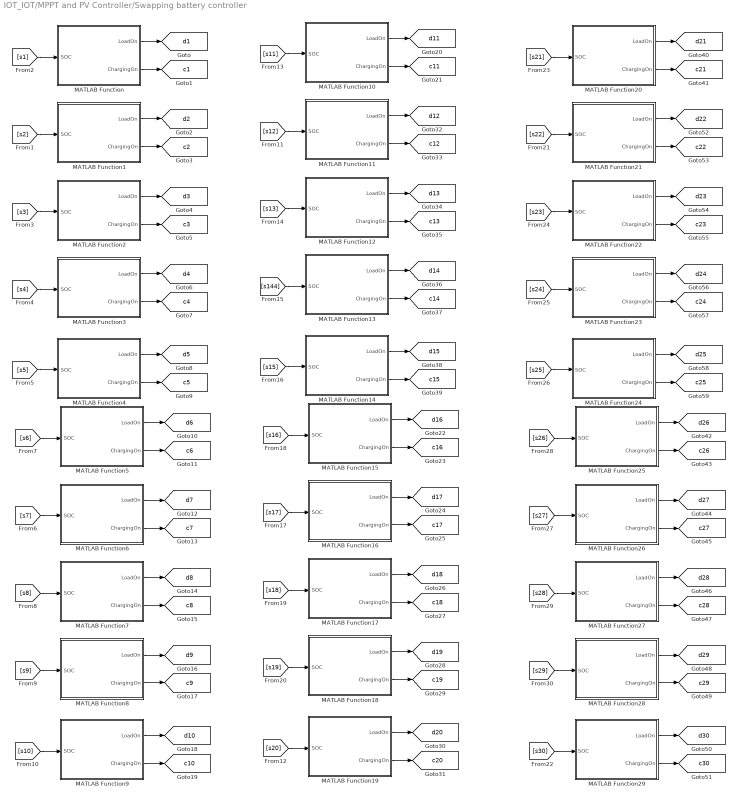
== system IOT_IOT/MPPT and PV Controller/Swapping battery controller ==
  MATLAB Function : MATLAB Function  TreatAsAtomicUnit=on
  MATLAB Function1 : MATLAB Function  TreatAsAtomicUnit=on
  MATLAB Function10 : MATLAB Function  TreatAsAtomicUnit=on
  MATLAB Function11 : MATLAB Function  TreatAsAtomicUnit=on
  MATLAB Function12 : MATLAB Function  TreatAsAtomicUnit=on
  MATLAB Function13 : MATLAB Function  TreatAsAtomicUnit=on
  MATLAB Function14 : MATLAB Function  TreatAsAtomicUnit=on
  MATLAB Function15 : MATLAB Function  TreatAsAtomicUnit=on
  MATLAB Function16 : MATLAB Function  TreatAsAtomicUnit=on
  MATLAB Function17 : MATLAB Function  TreatAsAtomicUnit=on
  MATLAB Function18 : MATLAB Function  TreatAsAtomicUnit=on
  MATLAB Function19 : MATLAB Function  TreatAsAtomicUnit=on
  MATLAB Function2 : MATLAB Function  TreatAsAtomicUnit=on
  MATLAB Function20 : MATLAB Function  TreatAsAtomicUnit=on
  MATLAB Function21 : MATLAB Function  TreatAsAtomicUnit=on
  MATLAB Function22 : MATLAB Function  TreatAsAtomicUnit=on
  MATLAB Function23 : MATLAB Function  TreatAsAtomicUnit=on
  MATLAB Function24 : MATLAB Function  TreatAsAtomicUnit=on
  MATLAB Function25 : MATLAB Function  TreatAsAtomicUnit=on
  MATLAB Function26 : MATLAB Function  TreatAsAtomicUnit=on
  MATLAB Function27 : MATLAB Function  TreatAsAtomicUnit=on
  MATLAB Function28 : MATLAB Function  TreatAsAtomicUnit=on
  MATLAB Function29 : MATLAB Function  TreatAsAtomicUnit=on
  MATLAB Function3 : MATLAB Function  TreatAsAtomicUnit=on
  MATLAB Function4 : MATLAB Function  TreatAsAtomicUnit=on
  MATLAB Function5 : MATLAB Function  TreatAsAtomicUnit=on
  MATLAB Function6 : MATLAB Function  TreatAsAtomicUnit=on
  MATLAB Function7 : MATLAB Function  TreatAsAtomicUnit=on
  MATLAB Function8 : MATLAB Function  TreatAsAtomicUnit=on
  MATLAB Function9 : MATLAB Function  TreatAsAtomicUnit=on
  tag scope: c10=global, c11=global, c12=global, c13=global, c14=global, c15=global, c16=global, c17=global, c18=global, c19=global, c1=global, c20=global, c21=global, c22=global, c23=global, c24=global, c25=global, c26=global, c27=global, c28=global, c29=global, c2=global, c30=global, c3=global, c4=global, c5=global, c6=global, c7=global, c8=global, c9=global, d10=global, d11=global, d12=global, d13=global, d14=global, d15=global, d16=global, d17=global, d18=global, d19=global, d1=global, d20=global, d21=global, d22=global, d23=global, d24=global, d25=global, d26=global, d27=global, d28=global, d29=global, d2=global, d30=global, d3=global, d4=global, d5=global, d6=global, d7=global, d8=global, d9=global
  wires:
  MATLAB Function10/1(LoadOn) -> [d11]
  MATLAB Function1/2(ChargingOn) -> [c2]
  [s20] -> MATLAB Function19/1(SOC)
  [s22] -> MATLAB Function21/1(SOC)
  MATLAB Function5/1(LoadOn) -> [d6]
  [s16] -> MATLAB Function15/1(SOC)
  [s5] -> MATLAB Function4/1(SOC)
  MATLAB Function/2(ChargingOn) -> [c1]
  MATLAB Function2/2(ChargingOn) -> [c3]
  MATLAB Function26/1(LoadOn) -> [d27]
  [s21] -> MATLAB Function20/1(SOC)
  MATLAB Function18/1(LoadOn) -> [d19]
  MATLAB Function7/2(ChargingOn) -> [c8]
  MATLAB Function12/2(ChargingOn) -> [c13]
  MATLAB Function28/1(LoadOn) -> [d29]
  MATLAB Function4/2(ChargingOn) -> [c5]
  MATLAB Function25/2(ChargingOn) -> [c26]
  [s1] -> MATLAB Function/1(SOC)
  MATLAB Function11/2(ChargingOn) -> [c12]
  MATLAB Function/1(LoadOn) -> [d1]
  MATLAB Function16/1(LoadOn) -> [d17]
  MATLAB Function10/2(ChargingOn) -> [c11]
  [s15] -> MATLAB Function14/1(SOC)
  [s12] -> MATLAB Function11/1(SOC)
  [s3] -> MATLAB Function2/1(SOC)
  MATLAB Function2/1(LoadOn) -> [d3]
  MATLAB Function17/1(LoadOn) -> [d18]
  MATLAB Function13/2(ChargingOn) -> [c14]
  MATLAB Function4/1(LoadOn) -> [d5]
  MATLAB Function14/2(ChargingOn) -> [c15]
  MATLAB Function3/1(LoadOn) -> [d4]
  MATLAB Function6/2(ChargingOn) -> [c7]
  [s7] -> MATLAB Function6/1(SOC)
  MATLAB Function15/1(LoadOn) -> [d16]
  MATLAB Function26/2(ChargingOn) -> [c27]
  [s8] -> MATLAB Function7/1(SOC)
  MATLAB Function6/1(LoadOn) -> [d7]
  MATLAB Function13/1(LoadOn) -> [d14]
  MATLAB Function16/2(ChargingOn) -> [c17]
  MATLAB Function18/2(ChargingOn) -> [c19]
  MATLAB Function5/2(ChargingOn) -> [c6]
  [s6] -> MATLAB Function5/1(SOC)
  [s18] -> MATLAB Function17/1(SOC)
  [s13] -> MATLAB Function12/1(SOC)
  MATLAB Function19/2(ChargingOn) -> [c20]
  MATLAB Function22/1(LoadOn) -> [d23]
  [s27] -> MATLAB Function26/1(SOC)
  MATLAB Function19/1(LoadOn) -> [d20]
  [s26] -> MATLAB Function25/1(SOC)
  [s29] -> MATLAB Function28/1(SOC)
  MATLAB Function8/2(ChargingOn) -> [c9]
  [s17] -> MATLAB Function16/1(SOC)
  MATLAB Function17/2(ChargingOn) -> [c18]
  [s19] -> MATLAB Function18/1(SOC)
  MATLAB Function3/2(ChargingOn) -> [c4]
  MATLAB Function11/1(LoadOn) -> [d12]
  [s11] -> MATLAB Function10/1(SOC)
  MATLAB Function8/1(LoadOn) -> [d9]
  [s2] -> MATLAB Function1/1(SOC)
  MATLAB Function12/1(LoadOn) -> [d13]
  [s10] -> MATLAB Function9/1(SOC)
  MATLAB Function14/1(LoadOn) -> [d15]
  [s144] -> MATLAB Function13/1(SOC)
  MATLAB Function1/1(LoadOn) -> [d2]
  [s4] -> MATLAB Function3/1(SOC)
  MATLAB Function15/2(ChargingOn) -> [c16]
  MATLAB Function7/1(LoadOn) -> [d8]
  [s9] -> MATLAB Function8/1(SOC)
  MATLAB Function9/1(LoadOn) -> [d10]
  MATLAB Function9/2(ChargingOn) -> [c10]
  MATLAB Function29/2(ChargingOn) -> [c30]
  MATLAB Function29/1(LoadOn) -> [d30]
  MATLAB Function27/2(ChargingOn) -> [c28]
  MATLAB Function25/1(LoadOn) -> [d26]
  [s28] -> MATLAB Function27/1(SOC)
  [s30] -> MATLAB Function29/1(SOC)
  MATLAB Function28/2(ChargingOn) -> [c29]
  MATLAB Function23/1(LoadOn) -> [d24]
  [s24] -> MATLAB Function23/1(SOC)
  MATLAB Function23/2(ChargingOn) -> [c24]
  MATLAB Function21/1(LoadOn) -> [d22]
  MATLAB Function27/1(LoadOn) -> [d28]
  MATLAB Function24/1(LoadOn) -> [d25]
  MATLAB Function22/2(ChargingOn) -> [c23]
  [s23] -> MATLAB Function22/1(SOC)
  MATLAB Function24/2(ChargingOn) -> [c25]
  [s25] -> MATLAB Function24/1(SOC)
  MATLAB Function20/2(ChargingOn) -> [c21]
  MATLAB Function21/2(ChargingOn) -> [c22]
  MATLAB Function20/1(LoadOn) -> [d21]

== system IOT_IOT/Scenario/Load switching ==
  Demux : Demux  Tag=STV Demux  Outputs=2
      settings: DisplayOption=none
  FromWs : FromWorkspace  Tag=STV FromWs  VariableName=tuvar
      SigBuilderData=|
      | common.afterFinalStr = 'Extrapolate'
      | common.sampleTime = 0
      | dataSet.timeRange = [0 10]
      | dataSet.name = 'Group 1'
      | sbobj.Groups.Name = 'Group 1'
      | sbobj.Groups.Signals(1).Name = 'Load 1'
      | sbobj.Groups.Signals(1).XData = [0 0.5 0.5 1.5 1.5 2.5 2.5 3.5 3.5 4 10]
      | sbobj.Groups.Signals(1).YData = [0 0 1 1 0 0 1 1 0 0 0]
      | sbobj.Groups.Signals(2).Name = 'Load 2'
      | sbobj.Groups.Signals(2).XData = [0 1 1 1.5 1.5 3 3 3.5 3.5 10]
      | sbobj.Groups.Signals(2).YData = [0 0 1 1 0 0 1 1 0 0]
  Load 1 : Outport  Tag=STV Outport  VectorParamsAs1DForOutWhenUnconnected=off
  Load 2 : Outport  Tag=STV Outport  Port=2  VectorParamsAs1DForOutWhenUnconnected=off
  wires:
  Demux/1 -> Load 1/1
  FromWs/1 -> Demux/1
  Demux/2 -> Load 2/1

== system IOT_IOT/Scenario/Power source ==
  Demux : Demux  Tag=STV Demux  Outputs=1
      settings: DisplayOption=none
  FromWs : FromWorkspace  Tag=STV FromWs  VariableName=tuvar
      SigBuilderData=|
      | common.afterFinalStr = 'Extrapolate'
      | common.sampleTime = 0
      | dataSet.timeRange = [0 10]
      | dataSet.name = 'Group 1'
      | sbobj.Groups.Name = 'Group 1'
      | sbobj.Groups.Signals.Name = 'Signal 2'
      | sbobj.Groups.Signals.XData = [0 2 2 4 4 10]
      | sbobj.Groups.Signals.YData = [1 1 0 0 1 1]
  Signal 2 : Outport  Tag=STV Outport  VectorParamsAs1DForOutWhenUnconnected=off
  wires:
  Demux/1 -> Signal 2/1
  FromWs/1 -> Demux/1

== system IOT_IOT/Solar/Irradiance  ==
  Demux : Demux  Tag=STV Demux  Outputs=2
      settings: DisplayOption=none
  FromWs : FromWorkspace  Tag=STV FromWs  VariableName=tuvar
      SigBuilderData=|
      | common.afterFinalStr = 'Extrapolate'
      | common.sampleTime = '0'
      | dataSet(1).timeRange = [0 2]
      | dataSet(1).name = 'Constant Irradiance'
      | dataSet(2).timeRange = [0 2]
      | dataSet(2).name = 'Step Irradiance'
      | dataSet(3).timeRange = [0 1]
      | dataSet(3).name = 'Ramp-up/down Irradiance'
      | sbobj.Groups(1).Name = 'Constant Irradiance'
      | sbobj.Groups(1).Signals(1).Name = 'Ir'
      | sbobj.Groups(1).Signals(1).XData = [0 2]
      | sbobj.Groups(1).Signals(1).YData = [1000 1000]
      | sbobj.Groups(1).Signals(2).Name = 'Temp'
      | sbobj.Groups(1).Signals(2).XData = [0 1 1 2]
      | sbobj.Groups(1).Signals(2).YData = [0 0 1 1]
      | sbobj.Groups(1).TimeRange = [0 2]
      | sbobj.Groups(2).Name = 'Step Irradiance'
      | sbobj.Groups(2).Signals(1).Name = 'Ir'
      | sbobj.Groups(2).Signals(1).XData = [0 0.252 0.252 2]
      | sbobj.Groups(2).Signals(1).YData = [600 600 1000 1000]
      | sbobj.Groups(2).Signals(2).Name = 'Temp'
      | sbobj.Groups(2).Signals(2).XData = [0 1 1 2]
      | sbobj.Groups(2).Signals(2).YData = [0 0 1 1]
      | sbobj.Groups(2).TimeRange = [0 2]
      | sbobj.Groups(3).Name = 'Ramp-up/down Irradiance'
      | sbobj.Groups(3).Signals(1).Name = 'Ir'
      | sbobj.Groups(3).Signals(1).XData = [0 0.3 0.3 0.4 0.4 0.5 0.5 1]
      | sbobj.Groups(3).Signals(1).YData = [1000 1000 800 795 600 600 400 395]
      | sbobj.Groups(3).Signals(2).Name = 'Temp'
      | sbobj.Groups(3).Signals(2).XData = [0 1]
      | sbobj.Groups(3).Signals(2).YData = [25 25]
      | sbobj.Groups(3).TimeRange = [0 1]
  Ir : Outport  Tag=STV Outport
  Temp : Outport  Tag=STV Outport  Port=2
  wires:
  Demux/1 -> Ir/1
  FromWs/1 -> Demux/1
  Demux/2 -> Temp/1

== system IOT_IOT/Solar/MPPT ==
  "V _ PV " : Inport
  I_PV : Inport  Port=2
  clock : Inport  Port=3
  Embedded MATLAB Function1 : MATLAB Function  TreatAsAtomicUnit=on
  Duty : Outport  VectorParamsAs1DForOutWhenUnconnected=off
  wires:
  Embedded MATLAB Function1/1(D) -> Duty/1
  clock/1 -> Embedded MATLAB Function1/3(T)
  "V _ PV "/1 -> Embedded MATLAB Function1/1(V)
  I_PV/1 -> Embedded MATLAB Function1/2(I)

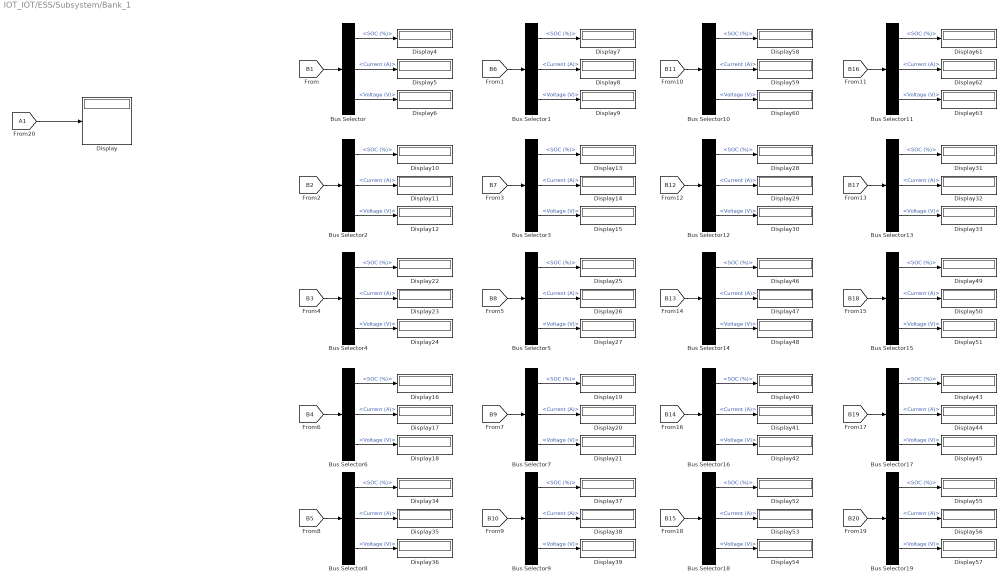
== system IOT_IOT/ESS/Subsystem/Bank_1 ==
  Bus Selector{,1..19} (20 alike) : BusSelector  OutputSignals=SOC (%),Current (A),Voltage (V)
  Display{,4..63} (61 alike) : Display
  wires:
  Bus Selector10/3 -> Display60/1  "<Voltage (V)>"
  Bus Selector4/2 -> Display23/1  "<Current (A)>"
  [B9] -> Bus Selector7/1
  Bus Selector7/3 -> Display21/1  "<Voltage (V)>"
  Bus Selector1/1 -> Display7/1  "<SOC (%)>"
  [B7] -> Bus Selector3/1
  Bus Selector16/3 -> Display42/1  "<Voltage (V)>"
  [B8] -> Bus Selector5/1
  Bus Selector17/1 -> Display43/1  "<SOC (%)>"
  Bus Selector1/2 -> Display8/1  "<Current (A)>"
  Bus Selector/3 -> Display6/1  "<Voltage (V)>"
  Bus Selector4/3 -> Display24/1  "<Voltage (V)>"
  [B4] -> Bus Selector6/1
  Bus Selector18/3 -> Display54/1  "<Voltage (V)>"
  [B19] -> Bus Selector17/1
  Bus Selector6/2 -> Display17/1  "<Current (A)>"
  Bus Selector/2 -> Display5/1  "<Current (A)>"
  [B3] -> Bus Selector4/1
  [B6] -> Bus Selector1/1
  Bus Selector12/3 -> Display30/1  "<Voltage (V)>"
  Bus Selector10/1 -> Display58/1  "<SOC (%)>"
  Bus Selector7/2 -> Display20/1  "<Current (A)>"
  Bus Selector6/1 -> Display16/1  "<SOC (%)>"
  Bus Selector16/2 -> Display41/1  "<Current (A)>"
  Bus Selector11/1 -> Display61/1  "<SOC (%)>"
  Bus Selector9/3 -> Display39/1  "<Voltage (V)>"
  Bus Selector3/2 -> Display14/1  "<Current (A)>"
  [B20] -> Bus Selector19/1
  Bus Selector5/2 -> Display26/1  "<Current (A)>"
  Bus Selector5/1 -> Display25/1  "<SOC (%)>"
  Bus Selector7/1 -> Display19/1  "<SOC (%)>"
  Bus Selector5/3 -> Display27/1  "<Voltage (V)>"
  Bus Selector4/1 -> Display22/1  "<SOC (%)>"
  Bus Selector9/1 -> Display37/1  "<SOC (%)>"
  Bus Selector2/3 -> Display12/1  "<Voltage (V)>"
  Bus Selector6/3 -> Display18/1  "<Voltage (V)>"
  [B17] -> Bus Selector13/1
  Bus Selector/1 -> Display4/1  "<SOC (%)>"
  Bus Selector1/3 -> Display9/1  "<Voltage (V)>"
  Bus Selector9/2 -> Display38/1  "<Current (A)>"
  Bus Selector17/2 -> Display44/1  "<Current (A)>"
  [B10] -> Bus Selector9/1
  Bus Selector8/1 -> Display34/1  "<SOC (%)>"
  Bus Selector11/3 -> Display63/1  "<Voltage (V)>"
  Bus Selector8/2 -> Display35/1  "<Current (A)>"
  Bus Selector8/3 -> Display36/1  "<Voltage (V)>"
  [B12] -> Bus Selector12/1
  [B2] -> Bus Selector2/1
  [B5] -> Bus Selector8/1
  Bus Selector2/2 -> Display11/1  "<Current (A)>"
  Bus Selector19/3 -> Display57/1  "<Voltage (V)>"
  Bus Selector3/3 -> Display15/1  "<Voltage (V)>"
  Bus Selector3/1 -> Display13/1  "<SOC (%)>"
  Bus Selector15/3 -> Display51/1  "<Voltage (V)>"
  [B11] -> Bus Selector10/1
  Bus Selector13/2 -> Display32/1  "<Current (A)>"
  [B15] -> Bus Selector18/1
  Bus Selector2/1 -> Display10/1  "<SOC (%)>"
  Bus Selector19/2 -> Display56/1  "<Current (A)>"
  [B1] -> Bus Selector/1
  Bus Selector12/1 -> Display28/1  "<SOC (%)>"
  Bus Selector12/2 -> Display29/1  "<Current (A)>"
  Bus Selector19/1 -> Display55/1  "<SOC (%)>"
  Bus Selector13/3 -> Display33/1  "<Voltage (V)>"
  Bus Selector13/1 -> Display31/1  "<SOC (%)>"
  Bus Selector18/1 -> Display52/1  "<SOC (%)>"
  Bus Selector18/2 -> Display53/1  "<Current (A)>"
  Bus Selector11/2 -> Display62/1  "<Current (A)>"
  Bus Selector15/1 -> Display49/1  "<SOC (%)>"
  Bus Selector14/1 -> Display46/1  "<SOC (%)>"
  Bus Selector14/3 -> Display48/1  "<Voltage (V)>"
  [B16] -> Bus Selector11/1
  Bus Selector15/2 -> Display50/1  "<Current (A)>"
  Bus Selector10/2 -> Display59/1  "<Current (A)>"
  [B14] -> Bus Selector16/1
  Bus Selector16/1 -> Display40/1  "<SOC (%)>"
  [B18] -> Bus Selector15/1
  [B13] -> Bus Selector14/1
  Bus Selector17/3 -> Display45/1  "<Voltage (V)>"
  Bus Selector14/2 -> Display47/1  "<Current (A)>"
  [A1] -> Display/1
